simulink model "FOC_MTPA"  (R2024b)
settings: Solver=ode4  StartTime=0.0  StopTime=100  FixedStep=10e-6  RelTol=1e-3
libraries: mcbcontrolslib x5, slpidlib x3, simulink x2, autolibpmsminterior x1
settings Model: Creator=Gokul-TRN0193  LastModifiedBy=Gokul-TRN0193
settings DebuggingCC: BusObjectLabelMismatch=error
settings RTWCC: Description=Create Visual C/C++ Solution File for Simulink Coder  TemplateMakefile=RTW.MSVCBuild
settings GRTTargetCC: MatFileLogging=off

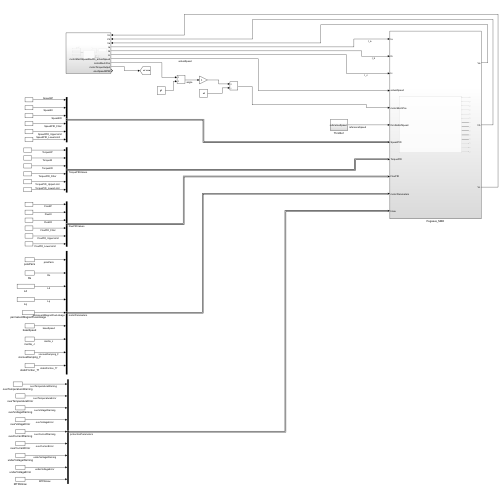
[thumbnail: Simulink's stored preview of the top-level diagram]
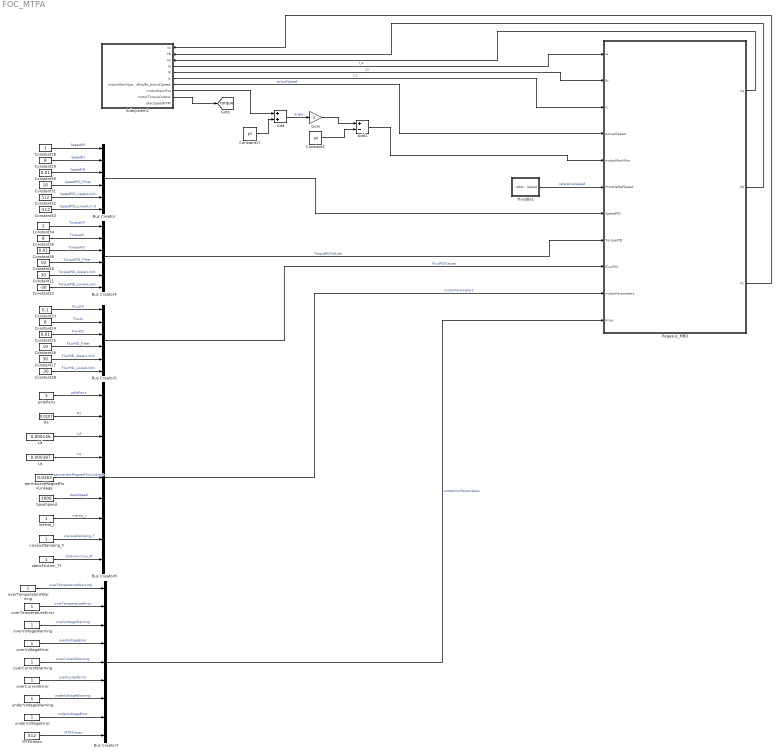
== system FOC_MTPA ==
  Add : Sum
  Add1 : Sum  Inputs=+-
  Bus Creator : BusCreator  Inputs=6
  Bus Creator4 : BusCreator  Inputs=6
  Bus Creator5 : BusCreator  Inputs=6
  Bus Creator7 : BusCreator  Inputs=9
  Bus Creator8 : BusCreator  Inputs=9
  Constant1 : Constant  Value=-pi  OutDataTypeStr=single
  Constant17 : Constant  Value=pi  OutDataTypeStr=single
  Constant19 : Constant
  Constant20 : Constant  Value=10
  Constant21 : Constant  Value=30
  Constant22 : Constant  Value=-30
  Constant23 : Constant  Value=0.1
  Constant24 : Constant  Value=8
  Constant25 : Constant  Value=0.01
  Constant26 : Constant  Value=10
  Constant27 : Constant  Value=30
  Constant28 : Constant  Value=-30
  Constant29 : Constant  Value=8
  Constant30 : Constant  Value=0.01
  Constant31 : Constant  Value=10
  Constant32 : Constant  Value=512
  Constant33 : Constant  Value=-512
  Constant34 : Constant  Value=2
  Constant35 : Constant  Value=8
  Constant36 : Constant  Value=0.01
  Gain : Gain  Gain=3
  Ld : Constant  Value=0.000146
  Lq : Constant  Value=0.000387
  MTPAImax : Constant  Value=512
  Pegasus_MBD : Subsystem
  Rs : Constant  Value=0.0107
  Subsystem1 : Subsystem
      settings: PortSchema="{\"entries\":[{\"content\":{\"sides\":[{\"content\":{},\"type\":\"ConnectorPlacement.EquallySpacedRectSide\",\"uuid\":\"d655f364-4693-4d11-886b-c83aead6f168\"},{\"content\":{\"connectorIds\":[\"In1\",\"In2\",\"In3\",\"Out1\",\"Out2\",\"Out3\",\"Out4\",\"Out5\",\"Out6\",\"Out7\"],\"side\":\"RIGHT\"},\"type\":\"ConnectorPlacement.EquallySpacedRectSide\",\"uuid\":\"4bb2d958-8bbb-488b-8d13-b01e05b3c8b3\"},{\"content\":{\"side\":\"TOP\"},\"type\":\"ConnectorPlacement.EquallySpacedRectSide\",\"uuid\":\"2f86fd26-f017-4c9e-8e6a-a37bffb400e3\"},{\"content\":{\"side\":\"BOTTOM\"},\"type\":\"ConnectorPlacement.EquallySpacedRectSide\",\"uuid\":\"ce04c704-7361-4f8c-8726-e9c60478a4f7\"}]},\"type\":\"ConnectorPlacement.EquallySpacedConnector\",\"uuid\":\"cd4018a2-c631-4ffc-af48-09e95c6f6864\"}],\"packageUris\":[\"http://schema.mathworks.com/mf0/Connector/R2020b\"],\"version\":\"1.0\"}"
  Throttle1 : Subsystem
  baseSpeed : Constant  Value=3000
  inertia_J : Constant
  overCurrentError : Constant
  overCurrentWarning : Constant
  overTemperatureError : Constant
  overTemperatureWarning : Constant
  overVoltageError : Constant
  overVoltageWarning : Constant
  permanentMagnetFluxLinkage : Constant  Value=0.0263
  polePairs : Constant  Value=3
  staticFriction_Tf : Constant
  underVoltageError : Constant
  underVoltageWarning : Constant
  viscousDamping_F : Constant
  tag scope: torque=global
  wires:
  Subsystem1/3(Ic) -> Pegasus_MBD/3(Ic)  "I_c"
  Pegasus_MBD/2(Vb) -> Subsystem1/2(Vb)
  Pegasus_MBD/3(Vc) -> Subsystem1/1(Vc)
  Throttle1/1(referenceSpeed) -> Pegasus_MBD/6(throttleRefSpeed)  "referenceSpeed"
  Subsystem1/1(Ia) -> Pegasus_MBD/1(Ia)  "I_a"
  Subsystem1/4(motorMechSpeedRadPs_actualSpeed) -> Pegasus_MBD/4(actualSpeed)  "actualSpeed"
  Subsystem1/2(Ib) -> Pegasus_MBD/2(Ib)  "I_b"
  Pegasus_MBD/1(Va) -> Subsystem1/3(Va)
  Bus Creator4/1 -> Pegasus_MBD/8(TorquePID)  "TorquePIDValues"
  Bus Creator5/1 -> Pegasus_MBD/9(FluxPID)  "FluxPIDValues"
  underVoltageWarning/1 -> Bus Creator7/7  "underVoltageWarning"
  overVoltageWarning/1 -> Bus Creator7/3  "overVoltageWarning"
  Constant27/1 -> Bus Creator5/5  "FluxPID_UpperLimit"
  Constant36/1 -> Bus Creator4/3  "TorqueKD"
  Bus Creator8/1 -> Pegasus_MBD/10(motorParameters)  "motorParameters"
  Constant20/1 -> Bus Creator4/4  "TorquePID_Filter"
  Constant25/1 -> Bus Creator5/3  "FluxKD"
  Constant35/1 -> Bus Creator4/2  "TorqueKI"
  Constant26/1 -> Bus Creator5/4  "FluxPID_Filter"
  Ld/1 -> Bus Creator8/3  "Ld"
  Constant23/1 -> Bus Creator5/1  "FluxKP"
  Constant21/1 -> Bus Creator4/5  "TorquePID_UpperLimit"
  overCurrentError/1 -> Bus Creator7/6  "overCurrentError"
  polePairs/1 -> Bus Creator8/1  "polePairs"
  viscousDamping_F/1 -> Bus Creator8/8  "viscousDamping_F"
  overVoltageError/1 -> Bus Creator7/4  "overVoltageError"
  inertia_J/1 -> Bus Creator8/7  "inertia_J"
  baseSpeed/1 -> Bus Creator8/6  "baseSpeed"
  Lq/1 -> Bus Creator8/4  "Lq"
  Constant22/1 -> Bus Creator4/6  "TorquePID_LowerLimit"
  overTemperatureError/1 -> Bus Creator7/2  "overTemperatureError"
  Bus Creator7/1 -> Pegasus_MBD/11(Imax)  "protectionParameters"
  Constant28/1 -> Bus Creator5/6  "FluxPID_LowerLimit"
  staticFriction_Tf/1 -> Bus Creator8/9  "staticFriction_Tf"
  overCurrentWarning/1 -> Bus Creator7/5  "overCurrentWarning"
  Constant24/1 -> Bus Creator5/2  "FluxKI"
  permanentMagnetFluxLinkage/1 -> Bus Creator8/5  "permanentMagnetFluxLinkage"
  overTemperatureWarning/1 -> Bus Creator7/1  "overTemperatureWarning"
  Constant34/1 -> Bus Creator4/1  "TorqueKP"
  underVoltageError/1 -> Bus Creator7/8  "underVoltageError"
  Rs/1 -> Bus Creator8/2  "Rs"
  MTPAImax/1 -> Bus Creator7/9  "MTPAImax"
  Constant32/1 -> Bus Creator/5  "SpeedPID_UpperLimit"
  Constant31/1 -> Bus Creator/4  "SpeedPID_Filter"
  Constant29/1 -> Bus Creator/2  "SpeedKI"
  Constant30/1 -> Bus Creator/3  "SpeedKD"
  Constant33/1 -> Bus Creator/6  "SpeedPID_LowerLimit"
  Constant19/1 -> Bus Creator/1  "SpeedKP"
  Bus Creator/1 -> Pegasus_MBD/7(SpeedPID)
  Subsystem1/6(motorTorqueOutput) -> [torque]
  Add1/1 -> Pegasus_MBD/5(motorMechPos)
  Add/1 -> Gain/1  "angle"
  Constant1/1 -> Add1/2
  Constant17/1 -> Add/2
  Subsystem1/5(motorMechPos) -> Add/1
  Gain/1 -> Add1/1

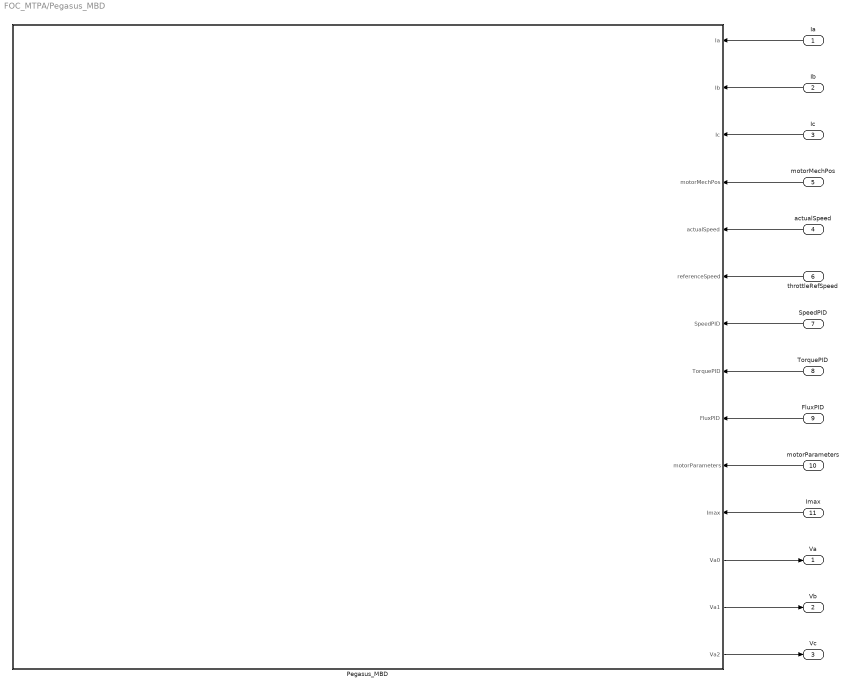
== system FOC_MTPA/Pegasus_MBD ==
  Ia : Inport
  Ib : Inport  Port=2
  Ic : Inport  Port=3
  actualSpeed : Inport  Port=4
  motorMechPos : Inport  Port=5
  throttleRefSpeed : Inport  Port=6
  SpeedPID : Inport  Port=7
  TorquePID : Inport  Port=8
  FluxPID : Inport  Port=9
  motorParameters : Inport  Port=10
  Imax : Inport  Port=11
  Pegasus_MBD : Subsystem
      settings: PortSchema="{\"entries\":[{\"content\":{\"sides\":[{\"content\":{},\"type\":\"ConnectorPlacement.EquallySpacedRectSide\",\"uuid\":\"6c18a17d-683c-442b-b8df-86db7e6c7e23\"},{\"content\":{\"connectorIds\":[\"In1\",\"In2\",\"In3\",\"In4\",\"In5\",\"In6\",\"In7\",\"In8\",\"In9\",\"In10\",\"In11\",\"Out1\",\"Out2\",\"Out3\"],\"side\":\"RIGHT\"},\"type\":\"ConnectorPlacement.EquallySpacedRectSide\",\"uuid\":\"c94cf015-fa73-4928-9364-a1e0e2fbcdea\"},{\"content\":{\"side\":\"TOP\"},\"type\":\"ConnectorPlacement.EquallySpacedRectSide\",\"uuid\":\"a268b29d-128b-4392-af37-e05faad43411\"}]},\"type\":\"ConnectorPlacement.EquallySpacedConnector\",\"uuid\":\"61323a96-d8bc-468c-bec5-27ea5f332e1f\"}],\"packageUris\":[\"http://schema.mathworks.com/mf0/Connector/R2020b\"],\"version\":\"1.0\"}"
  Va : Outport
  Vb : Outport  Port=2
  Vc : Outport  Port=3
  wires:
  Pegasus_MBD/3(Va2) -> Vc/1
  actualSpeed/1 -> Pegasus_MBD/5(actualSpeed)
  Ib/1 -> Pegasus_MBD/2(Ib)
  throttleRefSpeed/1 -> Pegasus_MBD/6(referenceSpeed)
  motorMechPos/1 -> Pegasus_MBD/4(motorMechPos)
  Pegasus_MBD/1(Va0) -> Va/1
  Ia/1 -> Pegasus_MBD/1(Ia)
  Pegasus_MBD/2(Va1) -> Vb/1
  Ic/1 -> Pegasus_MBD/3(Ic)
  SpeedPID/1 -> Pegasus_MBD/7(SpeedPID)
  TorquePID/1 -> Pegasus_MBD/8(TorquePID)
  FluxPID/1 -> Pegasus_MBD/9(FluxPID)
  motorParameters/1 -> Pegasus_MBD/10(motorParameters)
  Imax/1 -> Pegasus_MBD/11(Imax)

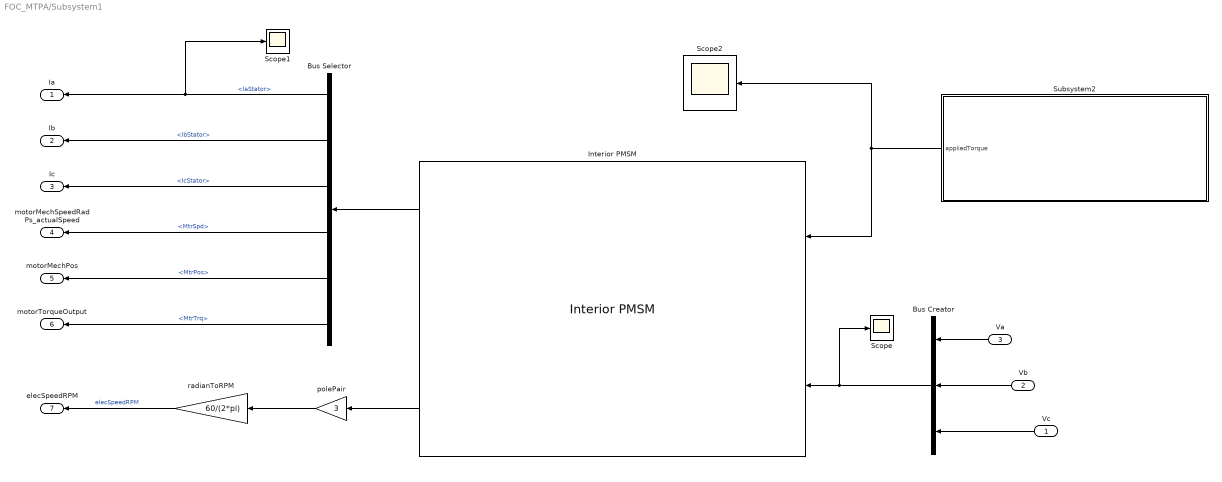
== system FOC_MTPA/Subsystem1 ==
  Vc : Inport
  Vb : Inport  Port=2
  Va : Inport  Port=3
  Bus Creator : BusCreator  Inputs=3
  Bus Selector : BusSelector  OutputSignals=IaStator,IbStator,IcStator,MtrSpd,MtrPos,MtrTrq
  Interior PMSM : autolibpmsminterior/Interior PMSM  port_config=Torque  sim_type=Continuous  Ts=0.001  P=3  Rs=0.0107  Ldq=[0.000146 0.000387]  KConstText=Permanent flux linkage constant (lambda_pm):  lambda_pm=0.0263  Ke=159.9771  mechanical=[0.004657,0.015,0.1]  idq0=[0 0]  theta_init=0  omega_init=0  KConst=0.0263  lambda_pm_calc=0.0263  Kt=0.07  RefBlkName='autolibpmsminterior/Interior PMSM'  aMode=5
  Scope : Scope
  Scope1 : Scope
  Scope2 : Scope
  Subsystem2 : Subsystem
  polePair : Gain  Gain=3
  radianToRPM : Gain  Gain=60/(2*pi)
  Ia : Outport
  Ib : Outport  Port=2
  Ic : Outport  Port=3
  motorMechSpeedRadPs_actualSpeed : Outport  Port=4
  motorMechPos : Outport  Port=5
  motorTorqueOutput : Outport  Port=6
  elecSpeedRPM : Outport  Port=7
  wires:
  Va/1 -> Bus Creator/1
  Bus Selector/4 -> motorMechSpeedRadPs_actualSpeed/1  "<MtrSpd>"
  Bus Selector/2 -> Ib/1  "<IbStator>"
  Vb/1 -> Bus Creator/2
  Interior PMSM/1 -> Bus Selector/1
  Subsystem2/1(appliedTorque) -> Interior PMSM/1, Scope2/1
  Vc/1 -> Bus Creator/3
  Interior PMSM/3 -> polePair/1
  Bus Selector/1 -> Scope1/1, Ia/1  "<IaStator>"
  Bus Selector/5 -> motorMechPos/1  "<MtrPos>"
  radianToRPM/1 -> elecSpeedRPM/1  "elecSpeedRPM"
  Bus Creator/1 -> Scope/1, Interior PMSM/2
  Bus Selector/6 -> motorTorqueOutput/1  "<MtrTrq>"
  polePair/1 -> radianToRPM/1
  Bus Selector/3 -> Ic/1  "<IcStator>"

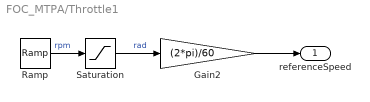
== system FOC_MTPA/Throttle1 ==
  Gain2 : Gain  Gain=(2*pi)/60
  Ramp : simulink/Sources/Ramp  slope=500  start=0  InitialOutput=0
  Saturation : Saturate  UpperLimit=2650
  referenceSpeed : Outport
  wires:
  Saturation/1 -> Gain2/1  "rad"
  Ramp/1 -> Saturation/1  "rpm"
  Gain2/1 -> referenceSpeed/1

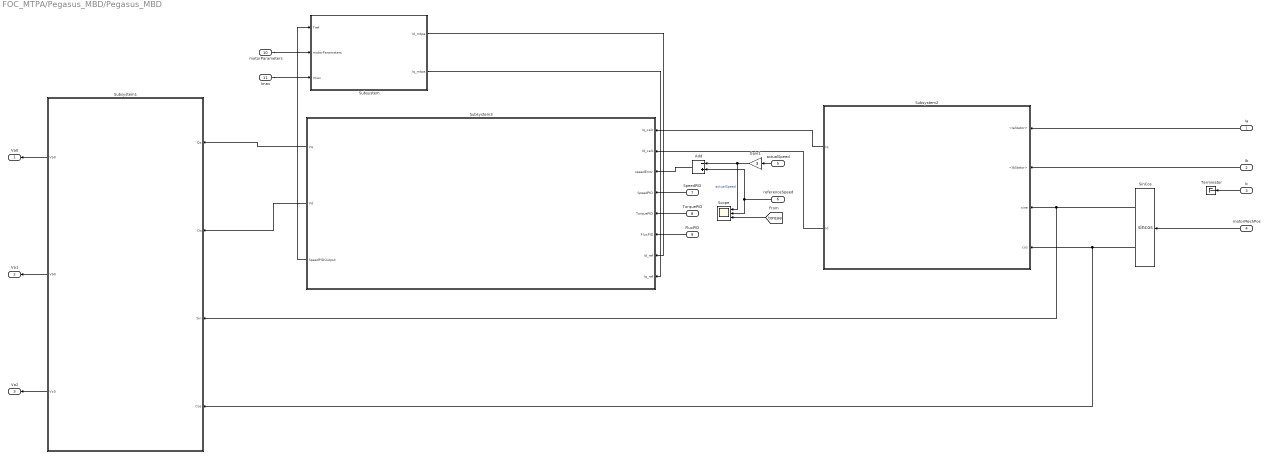
== system FOC_MTPA/Pegasus_MBD/Pegasus_MBD ==
  Ia : Inport
  Ib : Inport  Port=2
  Ic : Inport  Port=3
  motorMechPos : Inport  Port=4
  actualSpeed : Inport  Port=5
  referenceSpeed : Inport  Port=6
  SpeedPID : Inport  Port=7
  TorquePID : Inport  Port=8
  FluxPID : Inport  Port=9
  motorParameters : Inport  Port=10
  Imax : Inport  Port=11
  Add : Sum  Inputs=-+
  Gain1 : Gain  Gain=3
  Scope : Scope  NumInputPorts=3
  SinCos : Trigonometry  Operator=sincos
  Subsystem : Subsystem
  Subsystem1 : Subsystem
  Subsystem2 : Subsystem
  Subsystem3 : Subsystem
  Terminator : Terminator
  Va0 : Outport
  Va1 : Outport  Port=2
  Va2 : Outport  Port=3
  wires:
  SinCos/2 -> Subsystem1/4(Cos), Subsystem2/4(cos)
  SinCos/1 -> Subsystem1/3(Sin), Subsystem2/3(sine)
  Subsystem2/1(Iq) -> Subsystem3/1(Iq_calc)
  Subsystem2/2(Id) -> Subsystem3/2(Id_calc)
  Subsystem3/1(Vq) -> Subsystem1/1(Qs)
  Subsystem3/2(Vd) -> Subsystem1/2(Ds)
  Add/1 -> Subsystem3/3(speedError)
  Subsystem1/1(Va0) -> Va0/1
  Subsystem1/2(Vb0) -> Va1/1
  Subsystem1/3(Vc0) -> Va2/1
  Ia/1 -> Subsystem2/1(<IaStator>)
  Ib/1 -> Subsystem2/2(<IbStator>)
  motorMechPos/1 -> SinCos/1
  actualSpeed/1 -> Gain1/1
  Gain1/1 -> Add/1, Scope/1  "actualSpeed"
  referenceSpeed/1 -> Scope/2, Add/2
  Ic/1 -> Terminator/1
  SpeedPID/1 -> Subsystem3/4(SpeedPID)
  TorquePID/1 -> Subsystem3/5(TorquePID)
  FluxPID/1 -> Subsystem3/6(FluxPID)
  motorParameters/1 -> Subsystem/2(motorParameters)
  Imax/1 -> Subsystem/3(Imax)
  Subsystem3/3(SpeedPIDOutput) -> Subsystem/1(Tref)
  Subsystem/1(Id_mtpa) -> Subsystem3/7(Id_ref)
  Subsystem/2(Iq_mtpa) -> Subsystem3/8(Iq_ref)
  [torque] -> Scope/3

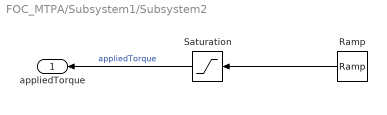
== system FOC_MTPA/Subsystem1/Subsystem2 ==
  Ramp : simulink/Sources/Ramp  slope=5  start=10  InitialOutput=0
  Saturation : Saturate  UpperLimit=50
  appliedTorque : Outport
  wires:
  Ramp/1 -> Saturation/1
  Saturation/1 -> appliedTorque/1  "appliedTorque"

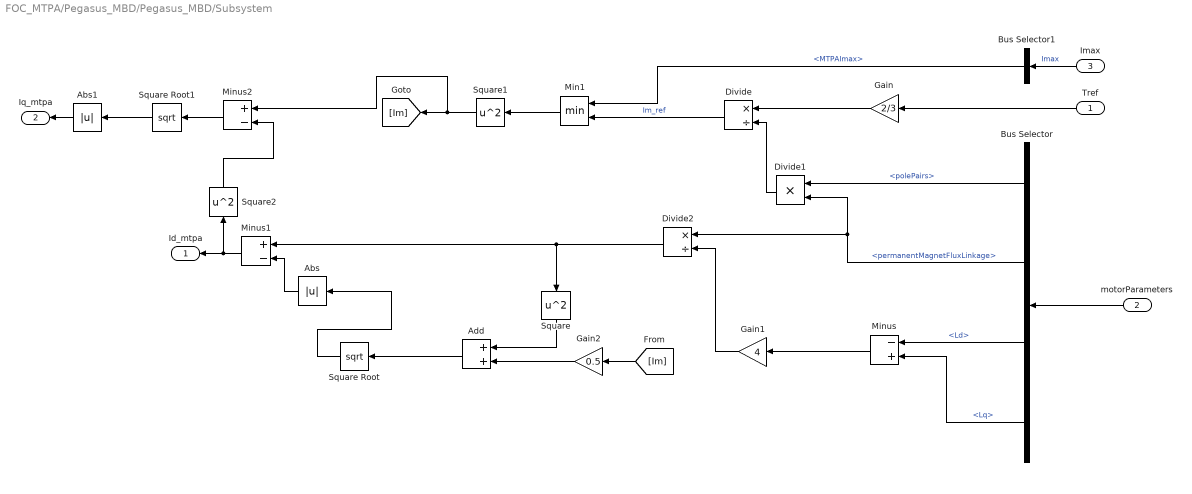
== system FOC_MTPA/Pegasus_MBD/Pegasus_MBD/Subsystem ==
  Tref : Inport
  motorParameters : Inport  Port=2
  Imax : Inport  Port=3
  Abs : Abs  SaturateOnIntegerOverflow=off
  Abs1 : Abs  SaturateOnIntegerOverflow=off
  Add : Sum
  Bus Selector : BusSelector  OutputSignals=polePairs,permanentMagnetFluxLinkage,Ld,Lq
  Bus Selector1 : BusSelector  OutputSignals=MTPAImax
  Divide : Product  Inputs=*/
  Divide1 : Product  Inputs=**
  Divide2 : Product  Inputs=*/
  Gain : Gain  Gain=2/3
  Gain1 : Gain  Gain=4
  Gain2 : Gain  Gain=0.5
  Min1 : MinMax  Inputs=2
  Minus : Sum  Inputs=-+
  Minus1 : Sum  Inputs=+-
  Minus2 : Sum  Inputs=+-
  Square : Math  Operator=square
  Square Root : Sqrt
  Square Root1 : Sqrt
  Square1 : Math  Operator=square
  Square2 : Math  Operator=square
  Id_mtpa : Outport
  Iq_mtpa : Outport  Port=2
  wires:
  Tref/1 -> Gain/1
  motorParameters/1 -> Bus Selector/1
  Gain/1 -> Divide/1
  Bus Selector/1 -> Divide1/1  "<polePairs>"
  Bus Selector/2 -> Divide1/2, Divide2/1  "<permanentMagnetFluxLinkage>"
  Divide1/1 -> Divide/2
  Divide/1 -> Min1/2  "Im_ref"
  Bus Selector/3 -> Minus/1  "<Ld>"
  Bus Selector/4 -> Minus/2  "<Lq>"
  Minus/1 -> Gain1/1
  Gain1/1 -> Divide2/2
  Divide2/1 -> Minus1/1, Square/1
  Square/1 -> Add/1
  Min1/1 -> Square1/1
  Square1/1 -> Minus2/1, [Im]
  [Im] -> Gain2/1
  Add/1 -> Square Root/1
  Square Root/1 -> Abs/1
  Abs/1 -> Minus1/2
  Minus1/1 -> Square2/1, Id_mtpa/1
  Gain2/1 -> Add/2
  Square2/1 -> Minus2/2
  Minus2/1 -> Square Root1/1
  Square Root1/1 -> Abs1/1
  Abs1/1 -> Iq_mtpa/1
  Imax/1 -> Bus Selector1/1  "Imax"
  Bus Selector1/1 -> Min1/1  "<MTPAImax>"

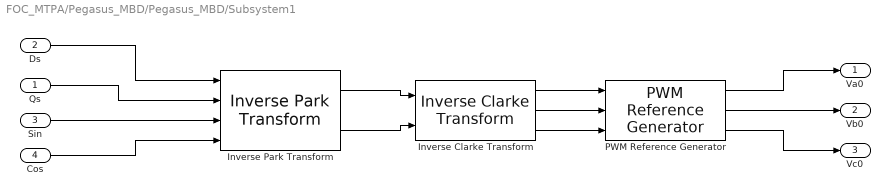
== system FOC_MTPA/Pegasus_MBD/Pegasus_MBD/Subsystem1 ==
  Qs : Inport
  Ds : Inport  Port=2
  Sin : Inport  Port=3
  Cos : Inport  Port=4
  Inverse Clarke Transform : mcbcontrolslib/Inverse Clarke Transform  PhaseInput=Two inputs  EnPowerInv=off
  Inverse Park Transform : mcbcontrolslib/Inverse Park Transform  PhaseInput=Two inputs  AxisAlignment=D-axis  ThetaInput=Sine and Cosine electrical position  AngleInput=Per-unit  N_points=1024
  PWM Reference Generator : mcbcontrolslib/PWM Reference Generator  inSignal=Vabc  modType=SVM: space vector modulation
  Va0 : Outport
  Vb0 : Outport  Port=2
  Vc0 : Outport  Port=3
  wires:
  Inverse Clarke Transform/3 -> PWM Reference Generator/3
  Ds/1 -> Inverse Park Transform/1
  Inverse Park Transform/2 -> Inverse Clarke Transform/2
  Cos/1 -> Inverse Park Transform/4
  Inverse Clarke Transform/2 -> PWM Reference Generator/2
  Inverse Park Transform/1 -> Inverse Clarke Transform/1
  Inverse Clarke Transform/1 -> PWM Reference Generator/1
  PWM Reference Generator/3 -> Vc0/1
  PWM Reference Generator/1 -> Va0/1
  Sin/1 -> Inverse Park Transform/3
  Qs/1 -> Inverse Park Transform/2
  PWM Reference Generator/2 -> Vb0/1

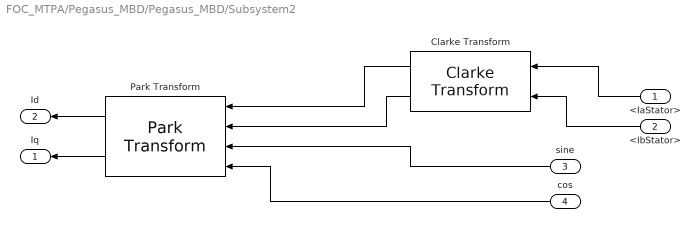
== system FOC_MTPA/Pegasus_MBD/Pegasus_MBD/Subsystem2 ==
  <IaStator> : Inport
  <IbStator> : Inport  Port=2
  sine : Inport  Port=3
  cos : Inport  Port=4
  Clarke Transform : mcbcontrolslib/Clarke Transform  VariantControl=Variant2  PhaseInput=Two inputs  EnPowerInv=off
  Park Transform : mcbcontrolslib/Park Transform  PhaseInput=Two inputs  AxisAlignment=D-axis  ThetaInput=Sine and Cosine electrical position  AngleInput=Per-unit  N_points=1024
  Iq : Outport
  Id : Outport  Port=2
  wires:
  Clarke Transform/1 -> Park Transform/1
  Clarke Transform/2 -> Park Transform/2
  sine/1 -> Park Transform/3
  cos/1 -> Park Transform/4
  <IaStator>/1 -> Clarke Transform/1
  <IbStator>/1 -> Clarke Transform/2
  Park Transform/1 -> Id/1
  Park Transform/2 -> Iq/1

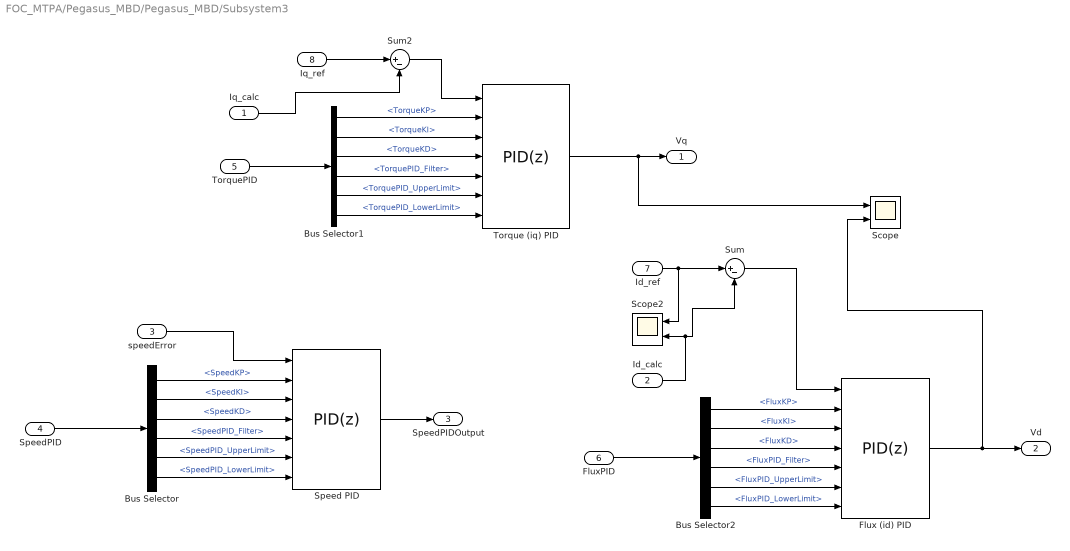
== system FOC_MTPA/Pegasus_MBD/Pegasus_MBD/Subsystem3 ==
  Iq_calc : Inport
  Id_calc : Inport  Port=2
  speedError : Inport  Port=3
  SpeedPID : Inport  Port=4
  TorquePID : Inport  Port=5
  FluxPID : Inport  Port=6
  Id_ref : Inport  Port=7
  Iq_ref : Inport  Port=8
  Bus Selector : BusSelector  OutputSignals=SpeedKP,SpeedKI,SpeedKD,SpeedPID_Filter,SpeedPID_UpperLimit,SpeedPID_LowerLimit
  Bus Selector1 : BusSelector  OutputSignals=TorqueKP,TorqueKI,TorqueKD,TorquePID_Filter,TorquePID_UpperLimit,TorquePID_LowerLimit
  Bus Selector2 : BusSelector  OutputSignals=FluxKP,FluxKI,FluxKD,FluxPID_Filter,FluxPID_UpperLimit,FluxPID_LowerLimit
  Flux (id) PID : slpidlib/PID Controller  Controller=PID  Form=Parallel  TimeDomain=Discrete-time  UseExternalTs=off  SampleTime=-1  IntegratorMethod=Forward Euler  FilterMethod=Forward Euler  ControllerParametersSource=external  P=1  I=1  UseKiTs=off  D=0  UseExternalDerivativeSource=off  N=100  UseFilter=on  TunerSelectOption=Transfer Function Based (PID Tuner App)  InitialConditionSource=internal  InitialConditionForIntegrator=0  InitialConditionForFilter=0  DifferentiatorICPrevScaledInput=0  ExternalReset=none  TrackingMode=off  Kt=1  LimitOutput=on  SatLimitsSource=external  UpperSaturationLimit=inf  LowerSaturationLimit=-inf  LinearizeAsGain=on  AntiWindupMode=clamping  Kb=1  LimitIntegrator=off  UpperIntegratorSaturationLimit=inf  LowerIntegratorSaturationLimit=-inf  POutMin=[]  POutMax=[]  IOutMin=[]  IOutMax=[]  DOutMin=[]  DOutMax=[]  NOutMin=[]  NOutMax=[]  SumOutMin=[]  SumOutMax=[]  SaturationOutMin=[]  SaturationOutMax=[]  PParamMin=[]  PParamMax=[]  IParamMin=[]  IParamMax=[]  DParamMin=[]  DParamMax=[]  NParamMin=[]  NParamMax=[]  KbParamMin=[]  KbParamMax=[]  KtParamMin=[]  KtParamMax=[]  KbOutMin=[]  KbOutMax=[]  KtOutMin=[]  KtOutMax=[]  IntegratorOutMin=[]  IntegratorOutMax=[]  FilterOutMin=[]  FilterOutMax=[]  SumI1OutMin=[]  SumI1OutMax=[]  SumI2OutMin=[]  SumI2OutMax=[]  SumI3OutMin=[]  SumI3OutMax=[]  SumI4OutMin=[]  SumI4OutMax=[]  SumDOutMin=[]  SumDOutMax=[]  DifferentiatorOutMin=[]  DifferentiatorOutMax=[]  FilterDiffOutCoefMin=[]  FilterDiffOutCoefMax=[]  ReciprocalOutMin=[]  ReciprocalOutMax=[]  SumDenOutMin=[]  SumDenOutMax=[]  SumNumOutMin=[]  SumNumOutMax=[]  DivideOutMin=[]  DivideOutMax=[]  UdiffTsProdOutMin=[]  UdiffTsProdOutMax=[]  NTsProdOutMin=[]  NTsProdOutMax=[]  UintegralTsProdOutMin=[]  UintegralTsProdOutMax=[]  UngainTsProdOutMin=[]  UngainTsProdOutMax=[]  ClampingZeroOutDataTypeStr=Inherit: Inherit via back propagation  ClampingZeroOutMin=[]  ClampingZeroOutMax=[]  FilterDenConstantOutDataTypeStr=Inherit: Inherit via back propagation  FilterDenConstantOutMin=[]  FilterDenConstantOutMax=[]  PCopyOutDataTypeStr=Inherit: Inherit via back propagation  PCopyOutMin=[]  PCopyOutMax=[]  NCopyOutDataTypeStr=Inherit: Inherit via back propagation  NCopyOutMin=[]  NCopyOutMax=[]  IntegratorContinuousStateAttributes=''  IntegratorStateMustResolveToSignalObject=off  IntegratorRTWStateStorageClass=Auto  FilterContinuousStateAttributes=''  FilterStateMustResolveToSignalObject=off  FilterRTWStateStorageClass=Auto  ParallelPVariant=ExternalParameters  IdealPVariant=Disabled  IVariant=ExternalParameters  DVariant=ExternalParameters  IntegratorVariant=Discrete  SatVariant=External  AWVariant=DiscClampingParallel  PCopyVariant=Disabled  TRVariant=Disabled  FdbkBlocksVariant=Forward  IdealPFdbkVariant=Disabled  SatFdbkVariant=Disabled  DerivativeFilterVariant=ForwardEulerFilter  NVariant=ExternalParameters  NCopyVariant=Disabled  FilterICVariant=InternalICsFilter  IntegratorICVariant=InternalICs  ExternalResetVariant=Disabled  TRSumVariant=Passthrough  SumFdbkVariant=Disabled  SumVariant=Sum_PID  TsampFilterVariant=InternalTs  TsampNgainVariant=Passthrough  TsampIntegralVariant=Disabled_SignalSpec  ExternalSaturationOutDataTypeStr=Inherit: Same as second input  DerivativeSourceVariant=ErrorSignal  PreIntVariant=InternalPreInt
  Scope : Scope  NumInputPorts=2
  Scope2 : Scope  NumInputPorts=2
  Speed PID : slpidlib/PID Controller  Controller=PID  Form=Parallel  TimeDomain=Discrete-time  UseExternalTs=off  SampleTime=-1  IntegratorMethod=Forward Euler  FilterMethod=Forward Euler  ControllerParametersSource=external  P=1  I=1  UseKiTs=off  D=0  UseExternalDerivativeSource=off  N=100  UseFilter=on  TunerSelectOption=Transfer Function Based (PID Tuner App)  InitialConditionSource=internal  InitialConditionForIntegrator=0  InitialConditionForFilter=0  DifferentiatorICPrevScaledInput=0  ExternalReset=none  TrackingMode=off  Kt=1  LimitOutput=on  SatLimitsSource=external  UpperSaturationLimit=inf  LowerSaturationLimit=-inf  LinearizeAsGain=on  AntiWindupMode=clamping  Kb=1  LimitIntegrator=off  UpperIntegratorSaturationLimit=inf  LowerIntegratorSaturationLimit=-inf  POutMin=[]  POutMax=[]  IOutMin=[]  IOutMax=[]  DOutMin=[]  DOutMax=[]  NOutMin=[]  NOutMax=[]  SumOutMin=[]  SumOutMax=[]  SaturationOutMin=[]  SaturationOutMax=[]  PParamMin=[]  PParamMax=[]  IParamMin=[]  IParamMax=[]  DParamMin=[]  DParamMax=[]  NParamMin=[]  NParamMax=[]  KbParamMin=[]  KbParamMax=[]  KtParamMin=[]  KtParamMax=[]  KbOutMin=[]  KbOutMax=[]  KtOutMin=[]  KtOutMax=[]  IntegratorOutMin=[]  IntegratorOutMax=[]  FilterOutMin=[]  FilterOutMax=[]  SumI1OutMin=[]  SumI1OutMax=[]  SumI2OutMin=[]  SumI2OutMax=[]  SumI3OutMin=[]  SumI3OutMax=[]  SumI4OutMin=[]  SumI4OutMax=[]  SumDOutMin=[]  SumDOutMax=[]  DifferentiatorOutMin=[]  DifferentiatorOutMax=[]  FilterDiffOutCoefMin=[]  FilterDiffOutCoefMax=[]  ReciprocalOutMin=[]  ReciprocalOutMax=[]  SumDenOutMin=[]  SumDenOutMax=[]  SumNumOutMin=[]  SumNumOutMax=[]  DivideOutMin=[]  DivideOutMax=[]  UdiffTsProdOutMin=[]  UdiffTsProdOutMax=[]  NTsProdOutMin=[]  NTsProdOutMax=[]  UintegralTsProdOutMin=[]  UintegralTsProdOutMax=[]  UngainTsProdOutMin=[]  UngainTsProdOutMax=[]  ClampingZeroOutDataTypeStr=Inherit: Inherit via back propagation  ClampingZeroOutMin=[]  ClampingZeroOutMax=[]  FilterDenConstantOutDataTypeStr=Inherit: Inherit via back propagation  FilterDenConstantOutMin=[]  FilterDenConstantOutMax=[]  PCopyOutDataTypeStr=Inherit: Inherit via back propagation  PCopyOutMin=[]  PCopyOutMax=[]  NCopyOutDataTypeStr=Inherit: Inherit via back propagation  NCopyOutMin=[]  NCopyOutMax=[]  IntegratorContinuousStateAttributes=''  IntegratorStateMustResolveToSignalObject=off  IntegratorRTWStateStorageClass=Auto  FilterContinuousStateAttributes=''  FilterStateMustResolveToSignalObject=off  FilterRTWStateStorageClass=Auto  ParallelPVariant=ExternalParameters  IdealPVariant=Disabled  IVariant=ExternalParameters  DVariant=ExternalParameters  IntegratorVariant=Discrete  SatVariant=External  AWVariant=DiscClampingParallel  PCopyVariant=Disabled  TRVariant=Disabled  FdbkBlocksVariant=Forward  IdealPFdbkVariant=Disabled  SatFdbkVariant=Disabled  DerivativeFilterVariant=ForwardEulerFilter  NVariant=ExternalParameters  NCopyVariant=Disabled  FilterICVariant=InternalICsFilter  IntegratorICVariant=InternalICs  ExternalResetVariant=Disabled  TRSumVariant=Passthrough  SumFdbkVariant=Disabled  SumVariant=Sum_PID  TsampFilterVariant=InternalTs  TsampNgainVariant=Passthrough  TsampIntegralVariant=Disabled_SignalSpec  ExternalSaturationOutDataTypeStr=Inherit: Same as second input  DerivativeSourceVariant=ErrorSignal  PreIntVariant=InternalPreInt
  Sum : Sum  Inputs=|+-
  Sum2 : Sum  Inputs=|+-
  Torque (iq) PID : slpidlib/PID Controller  Controller=PID  Form=Parallel  TimeDomain=Discrete-time  UseExternalTs=off  SampleTime=-1  IntegratorMethod=Forward Euler  FilterMethod=Forward Euler  ControllerParametersSource=external  P=1  I=1  UseKiTs=off  D=0  UseExternalDerivativeSource=off  N=100  UseFilter=on  TunerSelectOption=Transfer Function Based (PID Tuner App)  InitialConditionSource=internal  InitialConditionForIntegrator=0  InitialConditionForFilter=0  DifferentiatorICPrevScaledInput=0  ExternalReset=none  TrackingMode=off  Kt=1  LimitOutput=on  SatLimitsSource=external  UpperSaturationLimit=inf  LowerSaturationLimit=-inf  LinearizeAsGain=on  AntiWindupMode=clamping  Kb=1  LimitIntegrator=off  UpperIntegratorSaturationLimit=inf  LowerIntegratorSaturationLimit=-inf  POutMin=[]  POutMax=[]  IOutMin=[]  IOutMax=[]  DOutMin=[]  DOutMax=[]  NOutMin=[]  NOutMax=[]  SumOutMin=[]  SumOutMax=[]  SaturationOutMin=[]  SaturationOutMax=[]  PParamMin=[]  PParamMax=[]  IParamMin=[]  IParamMax=[]  DParamMin=[]  DParamMax=[]  NParamMin=[]  NParamMax=[]  KbParamMin=[]  KbParamMax=[]  KtParamMin=[]  KtParamMax=[]  KbOutMin=[]  KbOutMax=[]  KtOutMin=[]  KtOutMax=[]  IntegratorOutMin=[]  IntegratorOutMax=[]  FilterOutMin=[]  FilterOutMax=[]  SumI1OutMin=[]  SumI1OutMax=[]  SumI2OutMin=[]  SumI2OutMax=[]  SumI3OutMin=[]  SumI3OutMax=[]  SumI4OutMin=[]  SumI4OutMax=[]  SumDOutMin=[]  SumDOutMax=[]  DifferentiatorOutMin=[]  DifferentiatorOutMax=[]  FilterDiffOutCoefMin=[]  FilterDiffOutCoefMax=[]  ReciprocalOutMin=[]  ReciprocalOutMax=[]  SumDenOutMin=[]  SumDenOutMax=[]  SumNumOutMin=[]  SumNumOutMax=[]  DivideOutMin=[]  DivideOutMax=[]  UdiffTsProdOutMin=[]  UdiffTsProdOutMax=[]  NTsProdOutMin=[]  NTsProdOutMax=[]  UintegralTsProdOutMin=[]  UintegralTsProdOutMax=[]  UngainTsProdOutMin=[]  UngainTsProdOutMax=[]  ClampingZeroOutDataTypeStr=Inherit: Inherit via back propagation  ClampingZeroOutMin=[]  ClampingZeroOutMax=[]  FilterDenConstantOutDataTypeStr=Inherit: Inherit via back propagation  FilterDenConstantOutMin=[]  FilterDenConstantOutMax=[]  PCopyOutDataTypeStr=Inherit: Inherit via back propagation  PCopyOutMin=[]  PCopyOutMax=[]  NCopyOutDataTypeStr=Inherit: Inherit via back propagation  NCopyOutMin=[]  NCopyOutMax=[]  IntegratorContinuousStateAttributes=''  IntegratorStateMustResolveToSignalObject=off  IntegratorRTWStateStorageClass=Auto  FilterContinuousStateAttributes=''  FilterStateMustResolveToSignalObject=off  FilterRTWStateStorageClass=Auto  ParallelPVariant=ExternalParameters  IdealPVariant=Disabled  IVariant=ExternalParameters  DVariant=ExternalParameters  IntegratorVariant=Discrete  SatVariant=External  AWVariant=DiscClampingParallel  PCopyVariant=Disabled  TRVariant=Disabled  FdbkBlocksVariant=Forward  IdealPFdbkVariant=Disabled  SatFdbkVariant=Disabled  DerivativeFilterVariant=ForwardEulerFilter  NVariant=ExternalParameters  NCopyVariant=Disabled  FilterICVariant=InternalICsFilter  IntegratorICVariant=InternalICs  ExternalResetVariant=Disabled  TRSumVariant=Passthrough  SumFdbkVariant=Disabled  SumVariant=Sum_PID  TsampFilterVariant=InternalTs  TsampNgainVariant=Passthrough  TsampIntegralVariant=Disabled_SignalSpec  ExternalSaturationOutDataTypeStr=Inherit: Same as second input  DerivativeSourceVariant=ErrorSignal  PreIntVariant=InternalPreInt
  Vq : Outport
  Vd : Outport  Port=2
  SpeedPIDOutput : Outport  Port=3
  wires:
  Flux (id) PID/1 -> Scope/2, Vd/1
  Id_calc/1 -> Sum/2, Scope2/2
  Id_ref/1 -> Scope2/1, Sum/1
  Iq_calc/1 -> Sum2/2
  Sum/1 -> Flux (id) PID/1
  speedError/1 -> Speed PID/1
  Speed PID/1 -> SpeedPIDOutput/1
  Torque (iq) PID/1 -> Scope/1, Vq/1
  Bus Selector/2 -> Speed PID/3  "<SpeedKI>"
  Bus Selector/3 -> Speed PID/4  "<SpeedKD>"
  Bus Selector/4 -> Speed PID/5  "<SpeedPID_Filter>"
  Bus Selector/5 -> Speed PID/6  "<SpeedPID_UpperLimit>"
  Bus Selector/6 -> Speed PID/7  "<SpeedPID_LowerLimit>"
  Bus Selector1/1 -> Torque (iq) PID/2  "<TorqueKP>"
  Bus Selector1/2 -> Torque (iq) PID/3  "<TorqueKI>"
  Bus Selector1/3 -> Torque (iq) PID/4  "<TorqueKD>"
  Bus Selector1/4 -> Torque (iq) PID/5  "<TorquePID_Filter>"
  Bus Selector1/5 -> Torque (iq) PID/6  "<TorquePID_UpperLimit>"
  Bus Selector2/1 -> Flux (id) PID/2  "<FluxKP>"
  Bus Selector2/2 -> Flux (id) PID/3  "<FluxKI>"
  Bus Selector2/3 -> Flux (id) PID/4  "<FluxKD>"
  Bus Selector2/4 -> Flux (id) PID/5  "<FluxPID_Filter>"
  Bus Selector2/5 -> Flux (id) PID/6  "<FluxPID_UpperLimit>"
  Bus Selector2/6 -> Flux (id) PID/7  "<FluxPID_LowerLimit>"
  Bus Selector1/6 -> Torque (iq) PID/7  "<TorquePID_LowerLimit>"
  Bus Selector/1 -> Speed PID/2  "<SpeedKP>"
  SpeedPID/1 -> Bus Selector/1
  TorquePID/1 -> Bus Selector1/1
  FluxPID/1 -> Bus Selector2/1
  Sum2/1 -> Torque (iq) PID/1
  Iq_ref/1 -> Sum2/1
